simulink model "ThdRwLtStFwdBkwdSpdCtrl"  (R2018b)
settings: Solver=FixedStepDiscrete  StartTime=0.0  StopTime=10.0  FixedStep=0.01  RelTol=1e-3
libraries: simulink x6
settings Model: ModifiedHistory=2024.8.26 557无调速需求，发送默认值0  Creator=sn2xws  LastModifiedBy=sn2xws
settings DataIOCC: SaveFormat=StructureWithTime
settings OptimizationCC: DefaultParameterBehavior=Inlined  EnhancedBackFolding=on  PassReuseOutputArgsAs=Individual arguments  ZeroExternalMemoryAtStartup=off  ZeroInternalMemoryAtStartup=off  OptimizeBlockOrder=speed  DifferentSizesBufferReuse=on  OptimizationCustomize=off
settings DebuggingCC: ParameterTunabilityLossMsg=error
settings ModelReferenceCC: ModelReferenceNumInstancesAllowed=Single
settings SFSimCC: MATLABDynamicMemAlloc=off
settings RTWCC: SystemTargetFile=autosar.tlc  GenCodeOnly=on  TemplateMakefile=ert_default_tmf  Description=AUTOSAR  GenerateReport=on  IncludeHyperlinkInReport=on  LaunchReport=on  GenerateTraceInfo=on  GenerateTraceReport=on  GenerateTraceReportSl=on  GenerateTraceReportSf=on  GenerateTraceReportEml=on  GenerateCodeMetricsReport=on
settings CodeAppCC: ForceParamTrailComments=on  IgnoreCustomStorageClasses=off  OperatorAnnotations=on  SimulinkDataObjDesc=on  SFDataObjDesc=on  InsertBlockDesc=on
settings STFCustomTargetCC: TargetLangStandard=C99 (ISO)  MultiwordLength=256  ParMdlRefBuildCompliant=on  CompOptLevelCompliant=on  IncludeMdlTerminateFcn=off  CombineOutputUpdateFcns=on  SuppressErrorStatus=on  ERTCustomFileBanners=on  SupportNonFinite=off  SupportComplex=off  SupportContinuousTime=off  SupportNonInlinedSFcns=off  RemoveResetFunc=on  MATLABClassNameForMDSCustomization=Simulink.SoftwareTarget.ERTCustomization  AutosarCompliant=on  UseToolchainInfoCompliant=on  LookupTableObjectStructAxisOrder=2,1,3,4,...  LUTObjectStructOrderEvenSpacing=Size,Table,Breakpoints  SystemTargetFile=autosar.tlc
settings ERTTargetCC: TargetLangStandard=C99 (ISO)  ConcurrentExecutionCompliant=off  IncludeMdlTerminateFcn=off  SuppressErrorStatus=on  SupportNonFinite=off  SupportComplex=off  ModelStepFunctionPrototypeControlCompliant=off  CPPClassGenCompliant=off  AutosarCompliant=on  LookupTableObjectStructAxisOrder=2,1,3,4,...  LUTObjectStructOrderEvenSpacing=Size,Table,Breakpoints  InlinedParameterPlacement=NonHierarchical  ERTCustomFileTemplate=example_file_process.tlc  ERTFilePackagingFormat=Compact

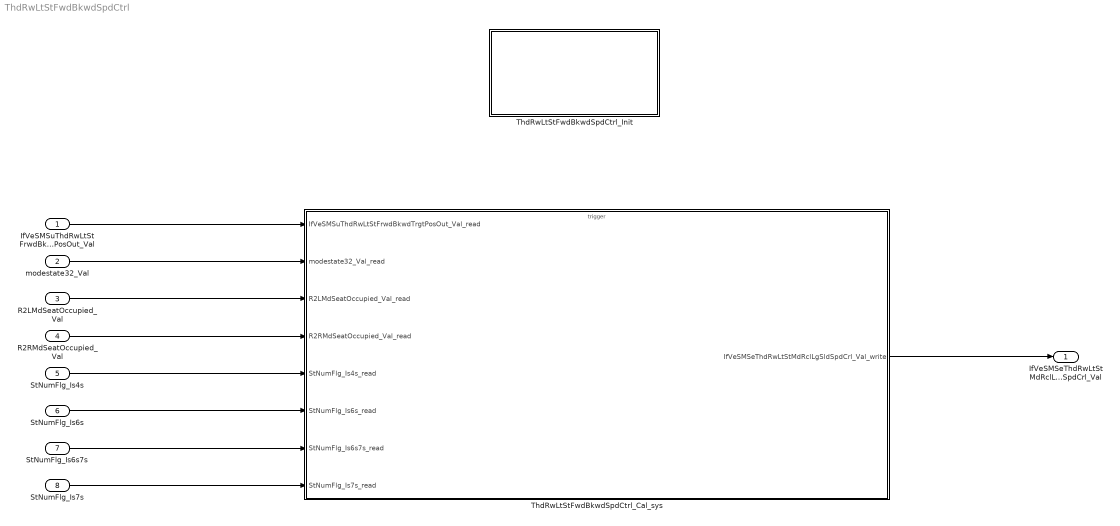
== system ThdRwLtStFwdBkwdSpdCtrl ==
  IfVeSMSuThdRwLtStFrwdBkwdTrgtPosOut_Val : Inport  OutDataTypeStr=boolean  PortDimensions=1
  modestate32_Val : Inport  Port=2  OutDataTypeStr=uint32  PortDimensions=1
  R2LMdSeatOccupied_Val : Inport  Port=3  OutDataTypeStr=boolean  PortDimensions=1
  R2RMdSeatOccupied_Val : Inport  Port=4  OutDataTypeStr=boolean  PortDimensions=1
  StNumFlg_Is4s : Inport  Port=5  OutDataTypeStr=boolean  PortDimensions=1
  StNumFlg_Is6s : Inport  Port=6  OutDataTypeStr=boolean  PortDimensions=1
  StNumFlg_Is6s7s : Inport  Port=7  OutDataTypeStr=boolean  PortDimensions=1
  StNumFlg_Is7s : Inport  Port=8  OutDataTypeStr=boolean  PortDimensions=1
  ThdRwLtStFwdBkwdSpdCtrl_Cal_sys : Subsystem
  ThdRwLtStFwdBkwdSpdCtrl_Init : Subsystem
  IfVeSMSeThdRwLtStMdRclLgSldSpdCrl_Val : Outport  OutDataTypeStr=uint8  PortDimensions=1
  wires:
  IfVeSMSuThdRwLtStFrwdBkwdTrgtPosOut_Val/1 -> ThdRwLtStFwdBkwdSpdCtrl_Cal_sys/1(IfVeSMSuThdRwLtStFrwdBkwdTrgtPosOut_Val_read)
  modestate32_Val/1 -> ThdRwLtStFwdBkwdSpdCtrl_Cal_sys/2(modestate32_Val_read)
  R2LMdSeatOccupied_Val/1 -> ThdRwLtStFwdBkwdSpdCtrl_Cal_sys/3(R2LMdSeatOccupied_Val_read)
  R2RMdSeatOccupied_Val/1 -> ThdRwLtStFwdBkwdSpdCtrl_Cal_sys/4(R2RMdSeatOccupied_Val_read)
  StNumFlg_Is4s/1 -> ThdRwLtStFwdBkwdSpdCtrl_Cal_sys/5(StNumFlg_Is4s_read)
  StNumFlg_Is6s/1 -> ThdRwLtStFwdBkwdSpdCtrl_Cal_sys/6(StNumFlg_Is6s_read)
  StNumFlg_Is6s7s/1 -> ThdRwLtStFwdBkwdSpdCtrl_Cal_sys/7(StNumFlg_Is6s7s_read)
  StNumFlg_Is7s/1 -> ThdRwLtStFwdBkwdSpdCtrl_Cal_sys/8(StNumFlg_Is7s_read)
  ThdRwLtStFwdBkwdSpdCtrl_Cal_sys/1(IfVeSMSeThdRwLtStMdRclLgSldSpdCrl_Val_write) -> IfVeSMSeThdRwLtStMdRclLgSldSpdCrl_Val/1

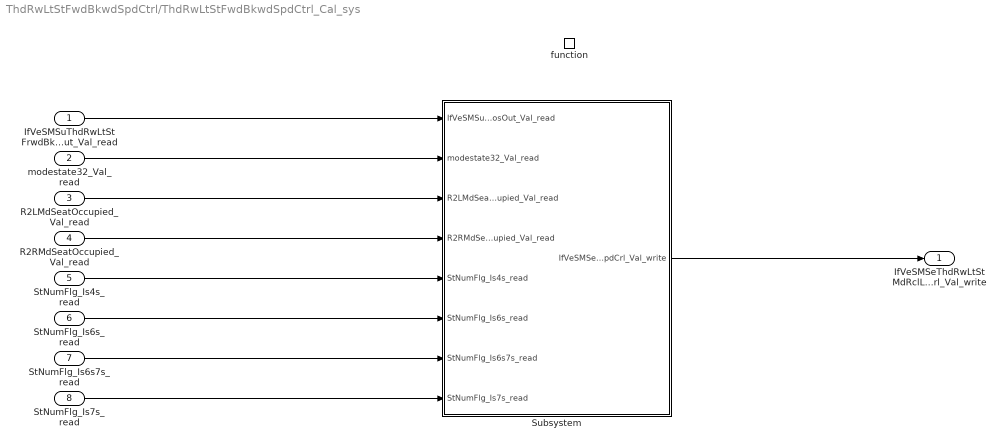
== system ThdRwLtStFwdBkwdSpdCtrl/ThdRwLtStFwdBkwdSpdCtrl_Cal_sys ==
  IfVeSMSuThdRwLtStFrwdBkwdTrgtPosOut_Val_read : Inport
  modestate32_Val_read : Inport  Port=2
  R2LMdSeatOccupied_Val_read : Inport  Port=3
  R2RMdSeatOccupied_Val_read : Inport  Port=4
  StNumFlg_Is4s_read : Inport  Port=5
  StNumFlg_Is6s_read : Inport  Port=6
  StNumFlg_Is6s7s_read : Inport  Port=7
  StNumFlg_Is7s_read : Inport  Port=8
  function : TriggerPort  TriggerType=function-call  IsSimulinkFunction=on  FunctionName=ThdRwLtStFwdBkwdSpdCtrl_Cal  VariantControl=(inherit)
  Subsystem : Subsystem
  IfVeSMSeThdRwLtStMdRclLgSldSpdCrl_Val_write : Outport
      settings: EnsureOutportIsVirtual=on
  wires:
  Subsystem/1(IfVeSMSeThdRwLtStMdRclLgSldSpdCrl_Val_write) -> IfVeSMSeThdRwLtStMdRclLgSldSpdCrl_Val_write/1
  R2RMdSeatOccupied_Val_read/1 -> Subsystem/4(R2RMdSeatOccupied_Val_read)
  StNumFlg_Is4s_read/1 -> Subsystem/5(StNumFlg_Is4s_read)
  IfVeSMSuThdRwLtStFrwdBkwdTrgtPosOut_Val_read/1 -> Subsystem/1(IfVeSMSuThdRwLtStFrwdBkwdTrgtPosOut_Val_read)
  modestate32_Val_read/1 -> Subsystem/2(modestate32_Val_read)
  R2LMdSeatOccupied_Val_read/1 -> Subsystem/3(R2LMdSeatOccupied_Val_read)
  StNumFlg_Is6s_read/1 -> Subsystem/6(StNumFlg_Is6s_read)
  StNumFlg_Is6s7s_read/1 -> Subsystem/7(StNumFlg_Is6s7s_read)
  StNumFlg_Is7s_read/1 -> Subsystem/8(StNumFlg_Is7s_read)

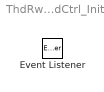
== system ThdRwLtStFwdBkwdSpdCtrl/ThdRwLtStFwdBkwdSpdCtrl_Init ==
  Event Listener : EventListener  EventName=reset

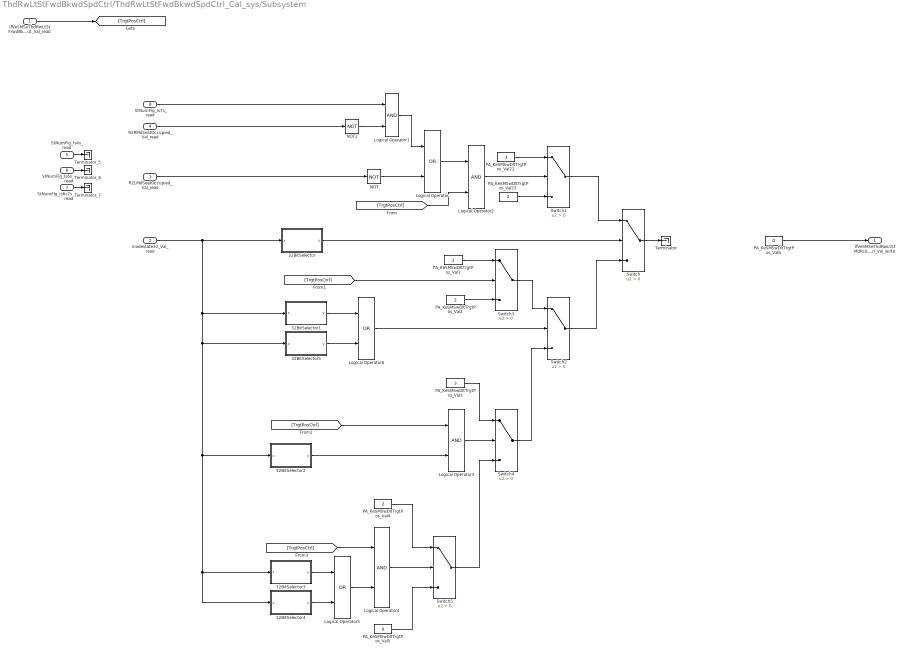
== system ThdRwLtStFwdBkwdSpdCtrl/ThdRwLtStFwdBkwdSpdCtrl_Cal_sys/Subsystem ==
  IfVeSMSuThdRwLtStFrwdBkwdTrgtPosOut_Val_read : Inport
  modestate32_Val_read : Inport  Port=2
  R2LMdSeatOccupied_Val_read : Inport  Port=3
  R2RMdSeatOccupied_Val_read : Inport  Port=4
  StNumFlg_Is4s_read : Inport  Port=5
  StNumFlg_Is6s_read : Inport  Port=6
  StNumFlg_Is6s7s_read : Inport  Port=7
  StNumFlg_Is7s_read : Inport  Port=8
  32BitSelector : Subsystem  mask(32 Bit Selector){BitNum=0}
      mask prompts: BitNum "Select Bit Number"
      mask help: Allows selection of a particular bit (0-31) out of a packed word up to 32 bits long. Output will be true if the bit number selected via the mask parameter is equal to one.
      mask TypeOptions BitNum: 0 | 1 | 2 | 3 | 4 | 5 | 6 | 7 | 8 | 9 | 10 | 11 | 12 | 13 | 14 | 15 | 16 | 17 | 18 | 19 | 20 | 21 | 22 | 23 | 24 | 25 | 26 | 27 | 28 | 29 | 30 | 31
      mask Display:
      | text(0.5, 0.8,'BIT','horizontalAlignment','center')
      | text(0.5, 0.5,'SELECTOR','horizontalAlignment','center')
      | text(0.5, 0.2,['-- Bit ',char(get_param(gcb,'BitNum')),' --'],'horizontalAlignment','center')
  32BitSelector1 : Subsystem  mask(32 Bit Selector){BitNum=9}
      mask prompts: BitNum "Select Bit Number"
      mask help: Allows selection of a particular bit (0-31) out of a packed word up to 32 bits long. Output will be true if the bit number selected via the mask parameter is equal to one.
      mask TypeOptions BitNum: 0 | 1 | 2 | 3 | 4 | 5 | 6 | 7 | 8 | 9 | 10 | 11 | 12 | 13 | 14 | 15 | 16 | 17 | 18 | 19 | 20 | 21 | 22 | 23 | 24 | 25 | 26 | 27 | 28 | 29 | 30 | 31
      mask Display:
      | text(0.5, 0.8,'BIT','horizontalAlignment','center')
      | text(0.5, 0.5,'SELECTOR','horizontalAlignment','center')
      | text(0.5, 0.2,['-- Bit ',char(get_param(gcb,'BitNum')),' --'],'horizontalAlignment','center')
  32BitSelector2 : Subsystem  mask(32 Bit Selector){BitNum=7}
      mask prompts: BitNum "Select Bit Number"
      mask help: Allows selection of a particular bit (0-31) out of a packed word up to 32 bits long. Output will be true if the bit number selected via the mask parameter is equal to one.
      mask TypeOptions BitNum: 0 | 1 | 2 | 3 | 4 | 5 | 6 | 7 | 8 | 9 | 10 | 11 | 12 | 13 | 14 | 15 | 16 | 17 | 18 | 19 | 20 | 21 | 22 | 23 | 24 | 25 | 26 | 27 | 28 | 29 | 30 | 31
      mask Display:
      | text(0.5, 0.8,'BIT','horizontalAlignment','center')
      | text(0.5, 0.5,'SELECTOR','horizontalAlignment','center')
      | text(0.5, 0.2,['-- Bit ',char(get_param(gcb,'BitNum')),' --'],'horizontalAlignment','center')
  32BitSelector3 : Subsystem  mask(32 Bit Selector){BitNum=6}
      mask prompts: BitNum "Select Bit Number"
      mask help: Allows selection of a particular bit (0-31) out of a packed word up to 32 bits long. Output will be true if the bit number selected via the mask parameter is equal to one.
      mask TypeOptions BitNum: 0 | 1 | 2 | 3 | 4 | 5 | 6 | 7 | 8 | 9 | 10 | 11 | 12 | 13 | 14 | 15 | 16 | 17 | 18 | 19 | 20 | 21 | 22 | 23 | 24 | 25 | 26 | 27 | 28 | 29 | 30 | 31
      mask Display:
      | text(0.5, 0.8,'BIT','horizontalAlignment','center')
      | text(0.5, 0.5,'SELECTOR','horizontalAlignment','center')
      | text(0.5, 0.2,['-- Bit ',char(get_param(gcb,'BitNum')),' --'],'horizontalAlignment','center')
  32BitSelector4 : Subsystem  mask(32 Bit Selector){BitNum=5}
      mask prompts: BitNum "Select Bit Number"
      mask help: Allows selection of a particular bit (0-31) out of a packed word up to 32 bits long. Output will be true if the bit number selected via the mask parameter is equal to one.
      mask TypeOptions BitNum: 0 | 1 | 2 | 3 | 4 | 5 | 6 | 7 | 8 | 9 | 10 | 11 | 12 | 13 | 14 | 15 | 16 | 17 | 18 | 19 | 20 | 21 | 22 | 23 | 24 | 25 | 26 | 27 | 28 | 29 | 30 | 31
      mask Display:
      | text(0.5, 0.8,'BIT','horizontalAlignment','center')
      | text(0.5, 0.5,'SELECTOR','horizontalAlignment','center')
      | text(0.5, 0.2,['-- Bit ',char(get_param(gcb,'BitNum')),' --'],'horizontalAlignment','center')
  32BitSelector5 : Subsystem  mask(32 Bit Selector){BitNum=11}
      mask prompts: BitNum "Select Bit Number"
      mask help: Allows selection of a particular bit (0-31) out of a packed word up to 32 bits long. Output will be true if the bit number selected via the mask parameter is equal to one.
      mask TypeOptions BitNum: 0 | 1 | 2 | 3 | 4 | 5 | 6 | 7 | 8 | 9 | 10 | 11 | 12 | 13 | 14 | 15 | 16 | 17 | 18 | 19 | 20 | 21 | 22 | 23 | 24 | 25 | 26 | 27 | 28 | 29 | 30 | 31
      mask Display:
      | text(0.5, 0.8,'BIT','horizontalAlignment','center')
      | text(0.5, 0.5,'SELECTOR','horizontalAlignment','center')
      | text(0.5, 0.2,['-- Bit ',char(get_param(gcb,'BitNum')),' --'],'horizontalAlignment','center')
  Logical Operator : Logic  Operator=OR  AllPortsSameDT=off  OutDataTypeStr=boolean
  Logical Operator{1..4} (4 alike) : Logic  AllPortsSameDT=off  OutDataTypeStr=boolean
  Logical Operator5 : Logic  Operator=OR  AllPortsSameDT=off  OutDataTypeStr=boolean
  Logical Operator6 : Logic  Operator=OR  AllPortsSameDT=off  OutDataTypeStr=boolean
  NOT : Logic  Operator=NOT  AllPortsSameDT=off  OutDataTypeStr=boolean
  NOT2 : Logic  Operator=NOT  AllPortsSameDT=off  OutDataTypeStr=boolean
  PA_KeSMSwDltTrgtPos_Val1 : Constant  Value=3  OutDataTypeStr=uint8
  PA_KeSMSwDltTrgtPos_Val2 : Constant  Value=2  OutDataTypeStr=uint8
  PA_KeSMSwDltTrgtPos_Val22 : Constant  Value=3  OutDataTypeStr=uint8
  PA_KeSMSwDltTrgtPos_Val23 : Constant  Value=2  OutDataTypeStr=uint8
  PA_KeSMSwDltTrgtPos_Val3 : Constant  Value=3  OutDataTypeStr=uint8
  PA_KeSMSwDltTrgtPos_Val4 : Constant  Value=2  OutDataTypeStr=uint8
  PA_KeSMSwDltTrgtPos_Val5 : Constant  Value=0  OutDataTypeStr=uint8
  PA_KeSMSwDltTrgtPos_Val6 : Constant  Value=0  OutDataTypeStr=uint8
  Switch{,1..5} (6 alike) : Switch  Criteria=u2 > Threshold
  Terminator : Terminator
  Terminator_5 : Terminator
  Terminator_6 : Terminator
  Terminator_7 : Terminator
  IfVeSMSeThdRwLtStMdRclLgSldSpdCrl_Val_write : Outport
      settings: EnsureOutportIsVirtual=on
  wires:
  modestate32_Val_read/1 -> 32BitSelector4/1(x), 32BitSelector3/1(x), 32BitSelector2/1(x), 32BitSelector5/1(x), 32BitSelector1/1(x), 32BitSelector/1(x)
  StNumFlg_Is6s_read/1 -> Terminator_6/1
  StNumFlg_Is6s7s_read/1 -> Terminator_7/1
  StNumFlg_Is4s_read/1 -> Terminator_5/1
  IfVeSMSuThdRwLtStFrwdBkwdTrgtPosOut_Val_read/1 -> [TrgtPosCtrl]
  [TrgtPosCtrl] -> Switch3/2
  NOT/1 -> Logical Operator/2
  PA_KeSMSwDltTrgtPos_Val1/1 -> Switch3/1
  32BitSelector2/1(y) -> Logical Operator3/2
  Logical Operator2/1 -> Switch1/2
  PA_KeSMSwDltTrgtPos_Val2/1 -> Switch3/3
  [TrgtPosCtrl] -> Logical Operator3/1
  StNumFlg_Is7s_read/1 -> Logical Operator1/1
  Logical Operator3/1 -> Switch4/2
  Switch4/1 -> Switch2/3
  PA_KeSMSwDltTrgtPos_Val23/1 -> Switch1/3
  NOT2/1 -> Logical Operator1/2
  R2RMdSeatOccupied_Val_read/1 -> NOT2/1
  Logical Operator4/1 -> Switch5/2
  Switch5/1 -> Switch4/3
  [TrgtPosCtrl] -> Logical Operator4/1
  PA_KeSMSwDltTrgtPos_Val4/1 -> Switch5/1
  PA_KeSMSwDltTrgtPos_Val3/1 -> Switch4/1
  Switch1/1 -> Switch/1
  PA_KeSMSwDltTrgtPos_Val5/1 -> Switch5/3
  Switch2/1 -> Switch/3
  [TrgtPosCtrl] -> Logical Operator2/2
  32BitSelector3/1(y) -> Logical Operator5/1
  Logical Operator1/1 -> Logical Operator/1
  PA_KeSMSwDltTrgtPos_Val22/1 -> Switch1/1
  Logical Operator5/1 -> Logical Operator4/2
  R2LMdSeatOccupied_Val_read/1 -> NOT/1
  Switch3/1 -> Switch2/1
  Logical Operator/1 -> Logical Operator2/1
  32BitSelector4/1(y) -> Logical Operator5/2
  32BitSelector/1(y) -> Switch/2
  32BitSelector1/1(y) -> Logical Operator6/1
  32BitSelector5/1(y) -> Logical Operator6/2
  Logical Operator6/1 -> Switch2/2
  Switch/1 -> Terminator/1
  PA_KeSMSwDltTrgtPos_Val6/1 -> IfVeSMSeThdRwLtStMdRclLgSldSpdCrl_Val_write/1

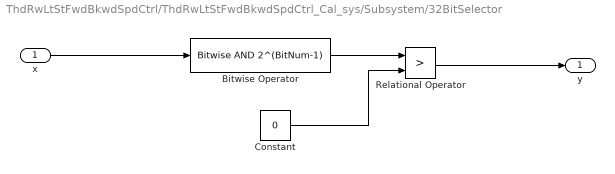
== system ThdRwLtStFwdBkwdSpdCtrl/ThdRwLtStFwdBkwdSpdCtrl_Cal_sys/Subsystem/32BitSelector ==
  x : Inport
  Bitwise Operator : simulink/Logic and Bit Operations/Bitwise Operator  logicop=AND  UseBitMask=on  BitMask=2^(BitNum-1)  BitMaskRealWorld=Stored Integer
  Constant : Constant  Value=0  OutDataTypeStr=uint32
  Relational Operator : RelationalOperator  Operator=>  OutDataTypeStr=boolean  RndMeth=Simplest
  y : Outport
  wires:
  Relational Operator/1 -> y/1
  Constant/1 -> Relational Operator/2
  x/1 -> Bitwise Operator/1
  Bitwise Operator/1 -> Relational Operator/1

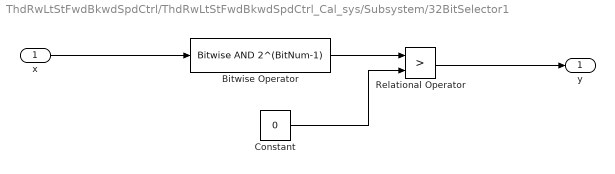
== system ThdRwLtStFwdBkwdSpdCtrl/ThdRwLtStFwdBkwdSpdCtrl_Cal_sys/Subsystem/32BitSelector1 ==
  x : Inport
  Bitwise Operator : simulink/Logic and Bit Operations/Bitwise Operator  logicop=AND  UseBitMask=on  BitMask=2^(BitNum-1)  BitMaskRealWorld=Stored Integer
  Constant : Constant  Value=0  OutDataTypeStr=uint32
  Relational Operator : RelationalOperator  Operator=>  OutDataTypeStr=boolean  RndMeth=Simplest
  y : Outport
  wires:
  Bitwise Operator/1 -> Relational Operator/1
  x/1 -> Bitwise Operator/1
  Constant/1 -> Relational Operator/2
  Relational Operator/1 -> y/1

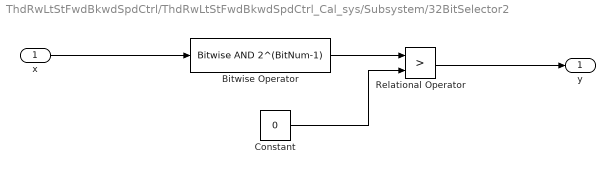
== system ThdRwLtStFwdBkwdSpdCtrl/ThdRwLtStFwdBkwdSpdCtrl_Cal_sys/Subsystem/32BitSelector2 ==
  x : Inport
  Bitwise Operator : simulink/Logic and Bit Operations/Bitwise Operator  logicop=AND  UseBitMask=on  BitMask=2^(BitNum-1)  BitMaskRealWorld=Stored Integer
  Constant : Constant  Value=0  OutDataTypeStr=uint32
  Relational Operator : RelationalOperator  Operator=>  OutDataTypeStr=boolean  RndMeth=Simplest
  y : Outport
  wires:
  Relational Operator/1 -> y/1
  Constant/1 -> Relational Operator/2
  x/1 -> Bitwise Operator/1
  Bitwise Operator/1 -> Relational Operator/1

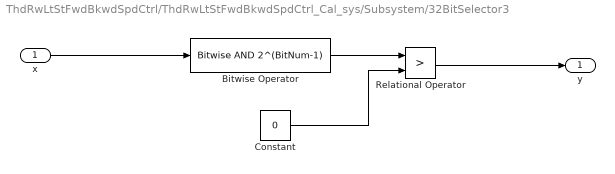
== system ThdRwLtStFwdBkwdSpdCtrl/ThdRwLtStFwdBkwdSpdCtrl_Cal_sys/Subsystem/32BitSelector3 ==
  x : Inport
  Bitwise Operator : simulink/Logic and Bit Operations/Bitwise Operator  logicop=AND  UseBitMask=on  BitMask=2^(BitNum-1)  BitMaskRealWorld=Stored Integer
  Constant : Constant  Value=0  OutDataTypeStr=uint32
  Relational Operator : RelationalOperator  Operator=>  OutDataTypeStr=boolean  RndMeth=Simplest
  y : Outport
  wires:
  Bitwise Operator/1 -> Relational Operator/1
  x/1 -> Bitwise Operator/1
  Constant/1 -> Relational Operator/2
  Relational Operator/1 -> y/1

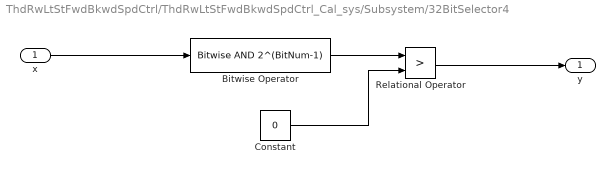
== system ThdRwLtStFwdBkwdSpdCtrl/ThdRwLtStFwdBkwdSpdCtrl_Cal_sys/Subsystem/32BitSelector4 ==
  x : Inport
  Bitwise Operator : simulink/Logic and Bit Operations/Bitwise Operator  logicop=AND  UseBitMask=on  BitMask=2^(BitNum-1)  BitMaskRealWorld=Stored Integer
  Constant : Constant  Value=0  OutDataTypeStr=uint32
  Relational Operator : RelationalOperator  Operator=>  OutDataTypeStr=boolean  RndMeth=Simplest
  y : Outport
  wires:
  Relational Operator/1 -> y/1
  Constant/1 -> Relational Operator/2
  x/1 -> Bitwise Operator/1
  Bitwise Operator/1 -> Relational Operator/1

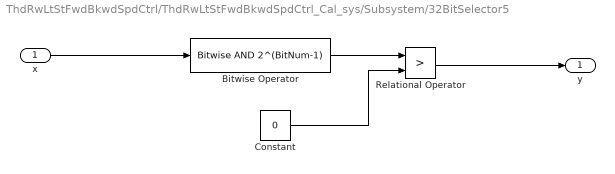
== system ThdRwLtStFwdBkwdSpdCtrl/ThdRwLtStFwdBkwdSpdCtrl_Cal_sys/Subsystem/32BitSelector5 ==
  x : Inport
  Bitwise Operator : simulink/Logic and Bit Operations/Bitwise Operator  logicop=AND  UseBitMask=on  BitMask=2^(BitNum-1)  BitMaskRealWorld=Stored Integer
  Constant : Constant  Value=0  OutDataTypeStr=uint32
  Relational Operator : RelationalOperator  Operator=>  OutDataTypeStr=boolean  RndMeth=Simplest
  y : Outport
  wires:
  Relational Operator/1 -> y/1
  Constant/1 -> Relational Operator/2
  x/1 -> Bitwise Operator/1
  Bitwise Operator/1 -> Relational Operator/1
